simulink model "StateAndSensorFaultEstim"  (R2025b)
settings: Solver=ode113  StartTime=0.0  StopTime=50  RelTol=1e-3
values from neighbouring files (symbols this model uses):
  hiddenLayerSizeFEstim = 3    [Init.m]
  hiddenLayerSizeObsv = 3    [Init.m]
  Vfestim0 = 0.1 * randn(hiddenLayerSizeFEstim, inputLayerSizeFEstim)    [Init.m]
  Vobsv0 = 0.1 * randn(hiddenLayerSizeObsv, inputLayerSizeObsv)    [Init.m]
  Wfestim0 = 0.1 * randn(outputLayerSizeFEstim, hiddenLayerSizeFEstim)    [Init.m]
  Wobsv0 = 0.1 * randn(outputLayerSizeObsv, hiddenLayerSizeObsv)    [Init.m]
undefined symbols (not defined in the file or in its folder): hiddenLayerSize, inputLayerSize, outputLayerSize
settings Model: Creator=Asus  LastModifiedBy=Asus

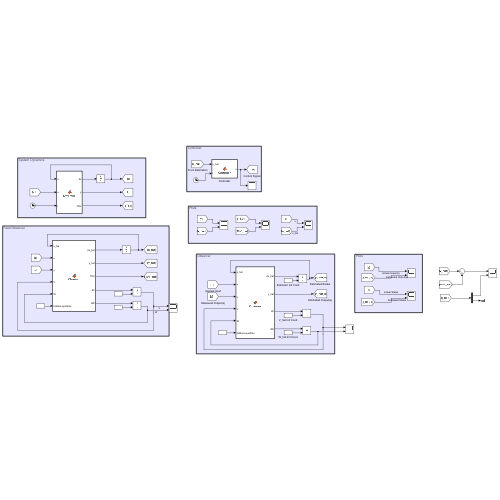
[thumbnail: Simulink's stored preview of the top-level diagram]
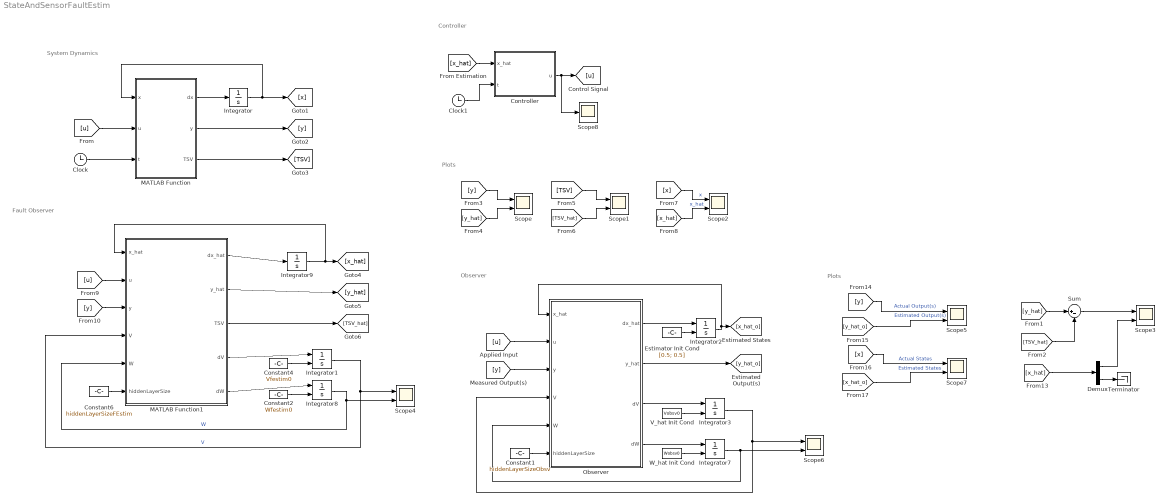
== system StateAndSensorFaultEstim ==
  note: System Dynamics
  note: Plots
  note: Fault Observer
  note: Plots
  note: Observer
  note: Controller
  Clock : Clock
  Clock1 : Clock
  Constant1 : Constant  Value=hiddenLayerSizeObsv
  Constant2 : Constant  Value=Wfestim0
  Constant4 : Constant  Value=Vfestim0
  Constant6 : Constant  Value=hiddenLayerSizeFEstim
  Controller : MATLAB Function  TreatAsAtomicUnit=on
  Demux : Demux  Outputs=2
  Estimator Init Cond : Constant  Value=[0.5; 0.5]
  Integrator : Integrator  InitialCondition=[0.5; 0.5]
  Integrator1 : Integrator  InitialConditionSource=external  InitialCondition=0.1 * randn(hiddenLayerSize, inputLayerSize)
  Integrator2 : Integrator  InitialConditionSource=external  InitialCondition=[0.5; 0.5]
  Integrator3 : Integrator  InitialConditionSource=external  InitialCondition=0.1 * randn(hiddenLayerSize, inputLayerSize)
  Integrator7 : Integrator  InitialConditionSource=external  InitialCondition=0.1 * randn(outputLayerSize, hiddenLayerSize)
  Integrator8 : Integrator  InitialConditionSource=external  InitialCondition=0.1 * randn(outputLayerSize, hiddenLayerSize)
  Integrator9 : Integrator  InitialCondition=[0.5; 0.5]
  MATLAB Function : MATLAB Function  TreatAsAtomicUnit=on
  MATLAB Function1 : MATLAB Function  TreatAsAtomicUnit=on
  Observer : MATLAB Function  TreatAsAtomicUnit=on
  Scope{,1..7} (8 alike) : Scope  NumInputPorts=2
      Scope settings: ActiveDisplayYMinimum=-5.00282570609E+6  ActiveDisplayYMaximum=4.502543135478E+7
      Scope1 settings: ActiveDisplayYMinimum=-0.81277488463586689  ActiveDisplayYMaximum=1.0445487559278768
      Scope2 settings: ActiveDisplayYMinimum=-0.12499999999999994  ActiveDisplayYMaximum=1.125  DataLoggingVariableName=ScopeData2
      Scope3 settings: ActiveDisplayYMinimum=-1  ActiveDisplayYMaximum=1
      Scope4 settings: ActiveDisplayYMinimum=-1  ActiveDisplayYMaximum=1  DataLoggingVariableName=ScopeData5
      Scope5 settings: ActiveDisplayYMinimum=-0.76155  ActiveDisplayYMaximum=1.44685
      Scope6 settings: ActiveDisplayYMinimum=-1.55238  ActiveDisplayYMaximum=1.13032  DataLoggingVariableName=ScopeData2
      Scope7 settings: ActiveDisplayYMinimum=-1  ActiveDisplayYMaximum=1  DataLoggingVariableName=ScopeData3
  Scope8 : Scope
      settings: ActiveDisplayYMinimum=-3.59635  ActiveDisplayYMaximum=2.36717  DataLoggingVariableName=ScopeData4
  Sum : Sum  Inputs=|+-
  Terminator : Terminator
  V_hat Init Cond : Constant  Value=Vobsv0
  W_hat Init Cond : Constant  Value=Wobsv0
  wires:
  [u] -> MATLAB Function/2(u)
  Clock/1 -> MATLAB Function/3(t)
  Integrator/1 -> MATLAB Function/1(x), [x]
  MATLAB Function/1(dx) -> Integrator/1
  MATLAB Function/2(y) -> [y]
  MATLAB Function/3(TSV) -> [TSV]
  [y] -> Scope/1
  [y_hat] -> Scope/2
  [TSV_hat] -> Scope1/2
  [TSV] -> Scope1/1
  [x_hat] -> Scope2/2  "x_hat"
  [x] -> Scope2/1  "x"
  [y_hat] -> Sum/1
  [TSV_hat] -> Sum/2
  Sum/1 -> Scope3/1
  [x_hat] -> Demux/1
  Demux/1 -> Scope3/2
  Demux/2 -> Terminator/1
  Clock1/1 -> Controller/2(t)
  [u] -> Observer/2(u)
  Observer/3(dV) -> Integrator3/1
  Estimator Init Cond/1 -> Integrator2/2
  W_hat Init Cond/1 -> Integrator7/2
  [y] -> Observer/3(y)
  Controller/1(u) -> [u], Scope8/1
  [x] -> Scope7/1  "Actual States"
  Observer/2(y_hat) -> [y_hat_o]
  Observer/1(dx_hat) -> Integrator2/1
  Observer/4(dW) -> Integrator7/1
  Integrator3/1 -> Scope6/1, Observer/4(V)
  [x_hat] -> Controller/1(x_hat)
  [x_hat_o] -> Scope7/2  "Estimated States"
  [y] -> Scope5/1  "Actual Output(s)"
  Integrator7/1 -> Scope6/2, Observer/5(W)
  Integrator2/1 -> Observer/1(x_hat), [x_hat_o]
  V_hat Init Cond/1 -> Integrator3/2
  [y_hat_o] -> Scope5/2  "Estimated Output(s)"
  Constant1/1 -> Observer/6(hiddenLayerSize)
  Constant2/1 -> Integrator8/2
  MATLAB Function1/4(dV) -> Integrator1/1
  Constant4/1 -> Integrator1/2
  MATLAB Function1/5(dW) -> Integrator8/1
  Integrator8/1 -> MATLAB Function1/5(W), Scope4/2  "W"
  Constant6/1 -> MATLAB Function1/6(hiddenLayerSize)
  Integrator1/1 -> Scope4/1, MATLAB Function1/4(V)  "V"
  MATLAB Function1/2(y_hat) -> [y_hat]
  MATLAB Function1/1(dx_hat) -> Integrator9/1
  MATLAB Function1/3(TSV) -> [TSV_hat]
  Integrator9/1 -> MATLAB Function1/1(x_hat), [x_hat]
  [u] -> MATLAB Function1/2(u)
  [y] -> MATLAB Function1/3(y)

== matlab function StateAndSensorFaultEstim/MATLAB Function1 ==
  data: x_hat input; u input; dx_hat output; y input; V input; W input; hiddenLayerSize input; y_hat output; TSV output; dV output; dW output
function [dx_hat, y_hat, TSV, dV, dW] = Observer(x_hat, u, y, V, W, hiddenLayerSize)
        
    fx_hat = [x_hat(2); x_hat(2) - x_hat(1)]; % f(x_hat)
    gx_hat = [0; 1];                % g(x_hat)
    C      = [1, 0];                % output matrix

    % designing params :
    Ac    = -1;
    eta   = 50 * [70; 70];
    gamma = 1  * [0.1; 0.1];

    % NN kernel function :
    kernel = @(phi) (-1 + 2 ./ (1 + exp(-2 * phi)));

    % designing observer :
    xNN = [x_hat; u];                      % NN inputs
    TSV = W' * kernel(V * xNN); % estimated sensor fault vector 

    % observer output :
    y_hat = C * x_hat + TSV;
    y_tilde   = y - y_hat;

    % observer derivative :
    dx_hat = fx_hat + gx_hat * u;

    % output layer weights adaption law :
    dW = - eta(1) * (y_tilde' * inv(Ac))' * kernel(V * xNN)' - gamma(1) * norm(y_tilde) * W'; %#ok
    % dW = zeros(size(W));

    % input layer weights adaption law :
    dV = - eta(2) * (y_tilde' * inv(Ac) * W' * (eye(hiddenLayerSize) - diag((kernel(V * xNN)).^2)))' * xNN' - gamma(2) * norm(y_tilde) * V; %#ok
    % dV = zeros(size(V));

end

== matlab function StateAndSensorFaultEstim/MATLAB Function ==
  data: x input; dx output; y output; u input; t input; TSV output
function [dx, y, TSV] = Dynamics(x, u, t)

    fx  = [x(2); x(2) - x(1)];
    gx  = [0; 1];               
    % TSV = 0 * (t > 5);         % sensor fault vector
    TSV = 1 * exp(-0.1*(t - 5)) * sin(t - 5) * (t > 5);         % sensor fault vector
    % TSV = 0;         % sensor fault vector
    C   = [1, 0];                % output matrix

    dx  = fx + gx * u;
    y   = C * x + TSV;

end

== matlab function StateAndSensorFaultEstim/Controller ==
  data: u output; x_hat input; t input
function u = Controller(x_hat, t)
    
    step = 1;
    k    = 4;
    u    = - [3, 5] * x_hat + k * step; % simple observer-based state feedback

end

== matlab function StateAndSensorFaultEstim/Observer ==
  data: dx_hat output; x_hat input; u input; y_hat output; y input; V input; W input; dV output; dW output; hiddenLayerSize input
function [dx_hat, y_hat, dV, dW] = Observer(x_hat, u, y, V, W, hiddenLayerSize)
    
    % arbitrary hurwitz matrix
    A = [0, 1; -1, -2];

    % system output matrix
    C = [1, 0];

    % observer gain
    G = [-19, 7]';

    % closed loop state matrix
    Ac = A - G * C;

    % designing params
    eta = 50 * [70; 70];
    rho = 1  * [0.1; 0.1];

    % hidden layer activation function
    kernel = @(z) (-1 + 2 ./ (1 + exp(-2 * z)));

    % neural network input
    xNN = [x_hat; u];

    % estimation of nonlinear terms
    g_hat  = W * kernel(V * xNN);
 
    % observer model
    dx_hat = A * x_hat + g_hat + G * (C * x_hat - y);
    y_hat  = C * x_hat;

    % observer error
    y_tilde = y_hat - y;

    % output layer weights adaption law
    dW = - eta(1) * (y_tilde' * C * inv(Ac))' * kernel(V * xNN)' - rho(1) * norm(y_tilde) * W; %#ok
    % dW = zeros(size(W));
    
    % input layer weights adaption law
    dV = - eta(2) * (y_tilde' * C * inv(Ac) * W * (eye(hiddenLayerSize) - diag((kernel(V * xNN)).^2)))' * tanh(xNN)' - rho(2) * norm(y_tilde) * V; %#ok
    % dV = zeros(size(V));
    
end
